simulink model "motion_complete"  (R2020a)
settings: Solver=VariableStepAuto  StartTime=0.0  StopTime=10.0  RelTol=1e-3
settings Model: Creator=simon  LastModifiedBy=simon

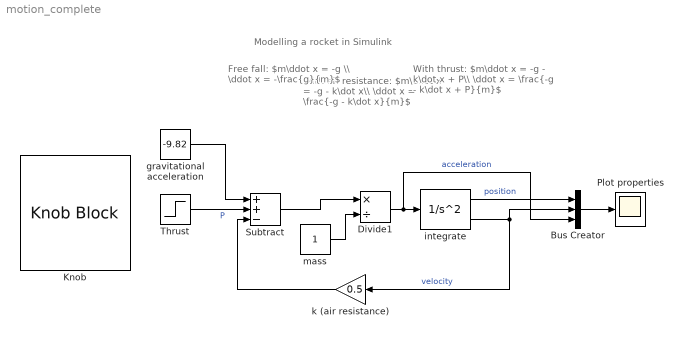
== system motion_complete ==
  note: Modelling a rocket in Simulink
  note: With air resistance:
      | $m\ddot x = -g - k\dot x\\ \ddot x = \frac{-g - k\dot x}{m}$
  note: Free fall:
      | $m\ddot x = -g \\ \ddot x = -\frac{g}{m}$
  note: With thrust:
      | $m\ddot x = -g - k\dot x + P\\ \ddot x = \frac{-g - k\dot x + P}{m}$
  Bus Creator : BusCreator  Inputs=3
  Divide1 : Product  Inputs=*/
  Knob : KnobBlock
  Plot properties : Scope
  Subtract : Sum  Inputs=++-
  Thrust : Step  Time=2  Before=30.92617797851563  After=0  SampleTime=0
  gravitational acceleration : Constant  Value=-9.82
  integrate : SecondOrderIntegrator  ICX=0
  k (air resistance) : Gain  Gain=0.5
  mass : Constant
  wires:
  gravitational acceleration/1 -> Subtract/1
  mass/1 -> Divide1/2
  integrate/2 -> Bus Creator/2, k (air resistance)/1  "velocity"
  Divide1/1 -> Bus Creator/3, integrate/1  "acceleration"
  integrate/1 -> Bus Creator/1  "position"
  k (air resistance)/1 -> Subtract/3
  Subtract/1 -> Divide1/1
  Bus Creator/1 -> Plot properties/1
  Thrust/1 -> Subtract/2  "P"
